simulink model "Robot_simulation"  (R2025b)
settings: Solver=VariableStepAuto  StartTime=0.0  StopTime=10  FixedStep=dt  RelTol=1e-3
InitFcn:
  | run("init.m");
values from neighbouring files (symbols this model uses):
  dt = 0.01    [init.m]
  F_max = 1500    [init.m]
  F_min = 100    [init.m]
  g = 9.81    [init.m]
  k_d = diag([5000, 5000])    [init.m]
  k_p = diag([20000, 20000])    [init.m]
  L_max = 0.8    [init.m]
  m3 = 60    [init.m]
  mb = 73    [init.m]
  mu = 0.6    [init.m]
  N = 15    [init.m]
  q_init = cinematica_inversa_2R(0, 0.6, robot_params)    [init.m]
  S_bar = 10*kron(eye(N), S)    [init.m]
  W_bar = kron(eye(N), W)    [init.m]
  x_ref = zeros(4, steps)    [init.m]
  x_ref_global = x_ref    [init.m]
  zb = 0.6    [init.m]
undefined symbols (not defined in the file or in its folder): DiscIntNeverNeededParam, robot_params
settings Model: Creator=Acer  LastModifiedBy=Acer

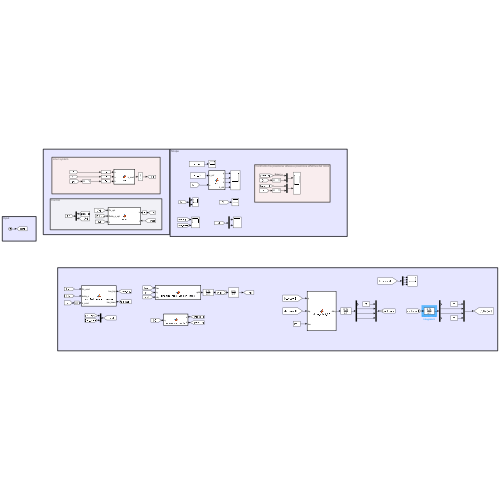
[thumbnail: Simulink's stored preview of the top-level diagram]
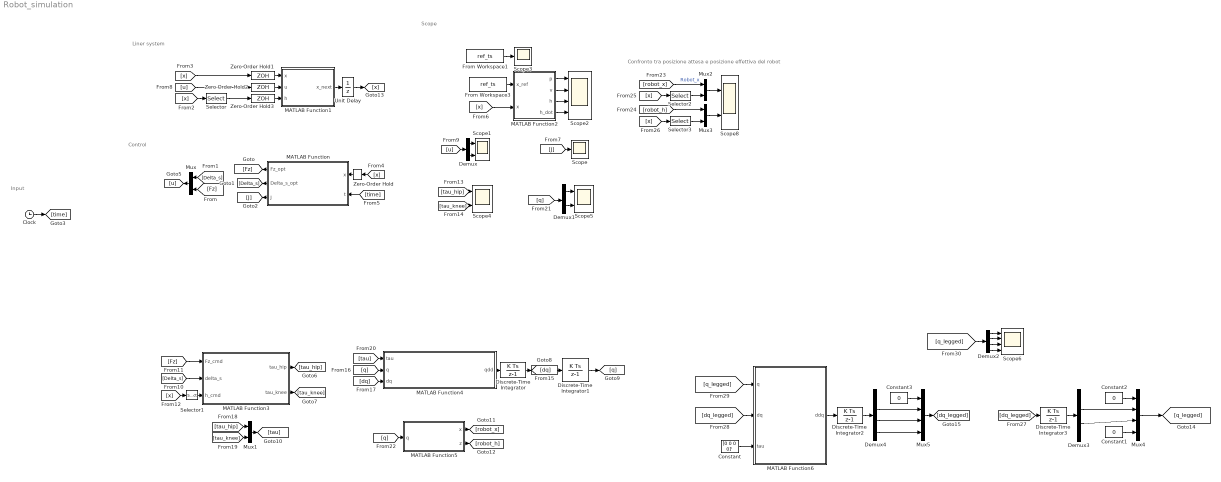
== system Robot_simulation ==
  note: Confronto tra posizione attesa e posizione effettiva del robot
  note: Control
  note: Liner system
  note: Input
  note: Scope
  Clock : Clock
  Constant : Constant  Value=[0 0 0 0]'
  Constant1 : Constant  Value=0
  Constant2 : Constant  Value=0
  Constant3 : Constant  Value=0
  Demux : Demux  Outputs=2
  Demux1 : Demux  Outputs=2
  Demux2 : Demux
  Demux3 : Demux
  Demux4 : Demux
  Discrete-Time Integrator : DiscreteIntegrator  InitialCondition=[0;0]  SampleTime=dt  ICPrevOutput=DiscIntNeverNeededParam  ICPrevScaledInput=DiscIntNeverNeededParam
  Discrete-Time Integrator1 : DiscreteIntegrator  InitialCondition=q_init  SampleTime=dt  ICPrevOutput=DiscIntNeverNeededParam  ICPrevScaledInput=DiscIntNeverNeededParam
  Discrete-Time Integrator2 : DiscreteIntegrator  InitialCondition=[0;0;0;0]  SampleTime=dt  ICPrevOutput=DiscIntNeverNeededParam  ICPrevScaledInput=DiscIntNeverNeededParam
  Discrete-Time Integrator3 : DiscreteIntegrator  InitialCondition=[0;-pi/2;0;0]  SampleTime=dt  ICPrevOutput=DiscIntNeverNeededParam  ICPrevScaledInput=DiscIntNeverNeededParam
  From Workspace1 : FromWorkspace  VariableName=ref_ts
  From Workspace3 : FromWorkspace  VariableName=ref_ts
  MATLAB Function : MATLAB Function  TreatAsAtomicUnit=on
  MATLAB Function1 : MATLAB Function  TreatAsAtomicUnit=on
  MATLAB Function2 : MATLAB Function  TreatAsAtomicUnit=on
  MATLAB Function3 : MATLAB Function  TreatAsAtomicUnit=on
  MATLAB Function4 : MATLAB Function  TreatAsAtomicUnit=on
  MATLAB Function5 : MATLAB Function  TreatAsAtomicUnit=on
  MATLAB Function6 : MATLAB Function  TreatAsAtomicUnit=on
  Mux{,1..3} (4 alike) : Mux  Inputs=2
  Mux4 : Mux
  Mux5 : Mux
  Scope : Scope
      settings: ActiveDisplayYMinimum=-1  ActiveDisplayYMaximum=1
  Scope{1,4..5,8} (4 alike) : Scope  NumInputPorts=2
      Scope1 settings: ActiveDisplayYMinimum=-0.020895768490500677  ActiveDisplayYMaximum=0.022328941684971165
      Scope4 settings: ActiveDisplayYMinimum=-14.847421541103996  ActiveDisplayYMaximum=15.870341136845298  DataLoggingVariableName=ScopeData4
      Scope5 settings: ActiveDisplayYMinimum=-1.7751159329900787E+253  ActiveDisplayYMaximum=1.5976043396910712E+254  DataLoggingVariableName=ScopeData5
      Scope8 settings: ActiveDisplayYMinimum=-0.36217276540062449  ActiveDisplayYMaximum=0.70314129266158121  DataLoggingVariableName=ScopeData8
  Scope2 : Scope  NumInputPorts=4
      settings: ActiveDisplayYMinimum=-0.12506830722069195  ActiveDisplayYMaximum=1.1256147649862278  DataLoggingVariableName=ScopeData2
  Scope3 : Scope
      settings: ActiveDisplayYMinimum=-1  ActiveDisplayYMaximum=1  DataLoggingVariableName=ScopeData3
  Scope6 : Scope  NumInputPorts=4
      settings: ActiveDisplayYMinimum=-1  ActiveDisplayYMaximum=1  DataLoggingVariableName=ScopeData6
  Selector : Selector  InputPortWidth=4  IndexOptions=Index vector (dialog)  Indices=[3]  OutputSizes=1
  Selector1 : Selector  InputPortWidth=4  IndexOptions=Index vector (dialog)  Indices=[3]  OutputSizes=1
  Selector2 : Selector  InputPortWidth=4  IndexOptions=Index vector (dialog)  Indices=1  OutputSizes=1
  Selector3 : Selector  InputPortWidth=4  IndexOptions=Index vector (dialog)  Indices=[3]  OutputSizes=1
  Unit Delay : UnitDelay  InitialCondition=x_ref(:,1)  SampleTime=-1  HasFrameUpgradeWarning=on
  Zero-Order Hold{,1..3} (4 alike) : ZeroOrderHold  SampleTime=dt
  wires:
  From Workspace1/1 -> Scope3/1
  MATLAB Function1/1(x_next) -> Unit Delay/1
  MATLAB Function/1(Fz_opt) -> [Fz]
  MATLAB Function/2(Delta_s_opt) -> [Delta_s]
  MATLAB Function/3(J) -> [J]
  Clock/1 -> [time]
  Unit Delay/1 -> [x]
  [Delta_s] -> Mux/1
  [Fz] -> Mux/2
  [x] -> Selector/1
  From Workspace3/1 -> MATLAB Function2/1(x_ref)
  MATLAB Function2/2(v) -> Scope2/2
  MATLAB Function2/1(p) -> Scope2/1
  MATLAB Function2/3(h) -> Scope2/3
  MATLAB Function2/4(h_dot) -> Scope2/4
  [x] -> MATLAB Function2/2(x)
  [J] -> Scope/1
  Mux/1 -> [u]
  [u] -> Demux/1
  Demux/1 -> Scope1/1
  Demux/2 -> Scope1/2
  [Delta_s] -> MATLAB Function3/2(delta_s)
  [Fz] -> MATLAB Function3/1(Fz_cmd)
  [x] -> Selector1/1
  Selector1/1 -> MATLAB Function3/3(h_cmd)
  MATLAB Function3/1(tau_hip) -> [tau_hip]
  MATLAB Function3/2(tau_knee) -> [tau_knee]
  [tau_knee] -> Scope4/2
  [tau_hip] -> Scope4/1
  MATLAB Function4/1(qdd) -> Discrete-Time Integrator/1
  Discrete-Time Integrator/1 -> [dq]
  [dq] -> Discrete-Time Integrator1/1
  Discrete-Time Integrator1/1 -> [q]
  [q] -> MATLAB Function4/2(q)
  [dq] -> MATLAB Function4/3(dq)
  [tau_hip] -> Mux1/1
  [tau_knee] -> Mux1/2
  Mux1/1 -> [tau]
  [tau] -> MATLAB Function4/1(tau)
  [q] -> Demux1/1
  Demux1/1 -> Scope5/1
  Demux1/2 -> Scope5/2
  MATLAB Function5/1(x) -> [robot_x]
  MATLAB Function5/2(z) -> [robot_h]
  [q] -> MATLAB Function5/1(q)
  [x] -> Selector2/1
  [x] -> Selector3/1
  [robot_x] -> Mux2/1  "Robot_x"
  Selector2/1 -> Mux2/2
  [robot_h] -> Mux3/1
  Selector3/1 -> Mux3/2
  Mux2/1 -> Scope8/1
  Mux3/1 -> Scope8/2
  Zero-Order Hold/1 -> MATLAB Function/1(x)
  [x] -> Zero-Order Hold/1
  [time] -> MATLAB Function/2(t)
  Constant/1 -> MATLAB Function6/3(tau)
  MATLAB Function6/1(ddq) -> Discrete-Time Integrator2/1
  [dq_legged] -> Discrete-Time Integrator3/1
  [q_legged] -> MATLAB Function6/1(q)
  Demux2/1 -> Scope6/1
  Demux2/2 -> Scope6/2
  Demux2/3 -> Scope6/3
  Demux2/4 -> Scope6/4
  [x] -> Zero-Order Hold1/1
  Zero-Order Hold1/1 -> MATLAB Function1/1(x)
  [u] -> Zero-Order Hold2/1
  Zero-Order Hold2/1 -> MATLAB Function1/2(u)
  Selector/1 -> Zero-Order Hold3/1
  Zero-Order Hold3/1 -> MATLAB Function1/3(h)
  [dq_legged] -> MATLAB Function6/2(dq)
  [q_legged] -> Demux2/1
  Constant1/1 -> Mux4/4
  Constant2/1 -> Mux4/1
  Discrete-Time Integrator3/1 -> Demux3/1
  Demux3/2 -> Mux4/2
  Demux3/3 -> Mux4/3
  Mux4/1 -> [q_legged]
  Discrete-Time Integrator2/1 -> Demux4/1
  Mux5/1 -> [dq_legged]
  Demux4/3 -> Mux5/3
  Constant3/1 -> Mux5/1
  Demux4/2 -> Mux5/2
  Demux4/4 -> Mux5/4

== matlab function Robot_simulation/MATLAB Function6 ==
  data: q input; ddq output size=4; dq input; tau input
function ddq =  whole_robot_2D(q, dq, tau)
    % tau è il vettore delle coppie/forze generalizzate in ingresso (4x1)
    
    % 1. Calcola le matrici dinamiche valutate nello stato attuale
    [M, C, G] = Dinamica_Robot(q, dq);
    
    % 2. Risolvi l'equazione del moto: M*ddq + C*dq + G = tau
    % In MATLAB/Simulink si usa l'operatore mldivide (\) per invertire M in modo robusto
    ddq = M \ (tau - C*dq - G);
end

== matlab function Robot_simulation/MATLAB Function1 ==
  data: x input size=4; x_next output size=4; u input size=2; h input size=1; g parameter; mb parameter; dt parameter
function x_next = fcn(x,u,h,g, mb,dt)

dc = [0; 0; 0; -g];     % Disturbo di gravità
dk = dc * dt;

Ac = [0 1 0 0; 0 0 0 0; 0 0 0 1; 0 0 0 0];
Bc = [0 0; g/h 0; 0 0; 0 1/mb];

    Ak = eye(4) + Ac * dt;
    Bk = Bc * dt;

   %dk disturbo di gravita
x_next = Ak*x + Bk*u + dk;

== matlab function Robot_simulation/MATLAB Function ==
  data: x input; Fz_opt output; t input; Delta_s_opt output; J output; zb parameter; g parameter; m3 parameter; dt parameter; mu parameter; W_bar parameter; S_bar parameter; F_max parameter; F_min parameter; N parameter; L_max parameter; x_ref_global parameter
function [Fz_opt, Delta_s_opt, J] = MPC(x,t,...              %INPUT
                                    zb, g, m3, dt, mu, W_bar, S_bar, F_max, F_min, N, L_max, x_ref_global) %PARAMETERS
% INPUT:
    % x_ref_global: Matrice intera della traiettoria [4 x steps]
    % t: Tempo di simulazione attuale (da un blocco Clock)

    % --- 1. GESTIONE DELLA TRAIETTORIA (SLIDING WINDOW) ---
    steps_totali = size(x_ref_global, 2);
    
    % Calcolo dell'indice attuale k basato sul tempo
    % Aggiungiamo 1 perché MATLAB usa indici che partono da 1 (t=0 -> k=1)
    k_curr = floor(t / dt) + 1; 
    
    % Inizializza il vettore per l'orizzonte N
    X_ref_window = zeros(4*N, 1);
    
    for i = 1:N
        % Calcola l'indice futuro. Il "min" serve come saturazione: 
        % se l'orizzonte guarda oltre la fine della simulazione, tiene l'ultimo target.
        idx = min(k_curr + i - 1, steps_totali); 
        
        % Inserisce i 4 stati futuri nello slot corretto
        X_ref_window((i-1)*4+1 : i*4) = x_ref_global(:, idx);
    end
    

    % INPUT: 
    % x_ref DEVE essere un vettore colonna [4*N x 1]. Se è una matrice, 
    % devi srotolarla prima di questa riga.

    h_k = x(3);
    dc = [0; 0; 0; -g];     % Disturbo di gravità
    dk = dc * dt;
    
    % --- Ricalcolo Dinamica Locale basata su h_k ---
    Ac = [0 1 0 0; 0 0 0 0; 0 0 0 1; 0 0 0 0];
    Bc = [0 0; g/h_k 0; 0 0; 0 1/m3];
    Ak = eye(4) + Ac * dt;
    Bk = Bc * dt;
    
    % --- Aggiornamento Dinamico dei Vincoli ---
    max_kinematic_ds = sqrt(L_max^2 - zb^2);
    ds_min = max(-mu*h_k, -max_kinematic_ds);
    ds_max = min(mu*h_k, max_kinematic_ds);
    
    U_min = [ds_min; F_min];
    U_max = [ds_max; F_max];
    LB = repmat(U_min, N, 1);
    UB = repmat(U_max, N, 1);
    
    % --- Calcolo Matrici di Predizione per l'orizzonte N ---
    Phi = zeros(4*N, 2*N);
    Psi = zeros(4*N, 4);
    Term_dist = zeros(4*N, 1);
    
    for i = 1:N
        Psi((i-1)*4+1:i*4, :) = Ak^i;
        for j = 1:i
            Phi((i-1)*4+1:i*4, (j-1)*2+1:j*2) = (Ak^(i-j)) * Bk;
            Term_dist((i-1)*4+1:i*4) = Term_dist((i-1)*4+1:i*4) + (Ak^(i-j))*dk;
        end
    end
    
    H = 2 * (Phi' * S_bar * Phi + W_bar);
    f = 2 * Phi' * S_bar * (Psi * x + Term_dist - X_ref_window);

 % --- 5. RISOLUZIONE QP ---
    options = optimoptions('quadprog', 'Algorithm', 'active-set', 'Display', 'off');
    
    % Definisci l'ingresso di equilibrio (Delta_s = 0, F_z = massa * gravità)
    u_guess_step = [0; m3* g];
    
    % Replicato per tutto l'orizzonte N
    U0_guess = repmat(u_guess_step, N, 1);
    
    % Passa U0_guess come 9° argomento invece di []
    [U_seq, fval, exitflag] = quadprog(H, f, [], [], [], [], LB, UB,U0_guess,options);
    
    % % --- Failsafe: Protezione contro il crash del solver ---
    % if exitflag <= 0 || isempty(U_seq)
    %     % Se fallisce, forza gli input a zero o a un valore di sicurezza
    %     U_seq = zeros(2*N, 1);
    %     fval = 0;
    % end
    
    % --- Calcolo del vero costo ---
    Errore_non_controllato = (Psi * x + Term_dist - X_ref_window);
    cost_costante = Errore_non_controllato' * S_bar * Errore_non_controllato;
    J = fval + cost_costante;
    
    % --- Assegnazione Output Corretta ---
    u_opt = U_seq(1:2);
    Delta_s_opt = u_opt(1); % u_1 controlla la dinamica x
    Fz_opt = u_opt(2);      % u_2 controlla la dinamica z

end

== matlab function Robot_simulation/MATLAB Function2 ==
  data: x_ref input; p output; x input; v output; h output; h_dot output
function [p, v, h, h_dot] = fcn(x_ref,x)

p = [x_ref(1),x(1)];
v = [x_ref(2),x(2)];
h = [x_ref(3),x(3)];
h_dot = [x_ref(4),x(4)];

== matlab function Robot_simulation/MATLAB Function3 ==
  data: Fz_cmd input; tau_hip output; delta_s input; h_cmd input; k_p parameter; k_d parameter; tau_knee output; robot_params parameter
function [tau_hip, tau_knee] = new_Task_space_controller(Fz_cmd, delta_s, h_cmd, k_p, k_d, robot_params)
    %% 1. Cinematica Inversa (IK) - Modello D-H Standard
    % Target: [delta_s; h_cmd] (posizione end-effector)
    % L'ipotenusa L

    l1 = robot_params.l1;
    l2 = robot_params.l2;

    dist_sq = delta_s^2 + h_cmd^2;
    L = sqrt(dist_sq);
    
    % Legge del coseno per q2 (relativo)
    cos_q2 = (dist_sq - l1^2 - l2^2) / (2 * l1 * l2);
    cos_q2 = max(min(cos_q2, 1), -1); % Saturazione numerica
    q2 = acos(cos_q2); % Configurazione: ginocchio flesso positivo
    
    % Angolo q1 (anca)
    q1 = atan2(h_cmd, delta_s) - atan2(l2*sin(q2), l1 + l2*cos(q2));
    
    %% 2. Jacobiano Analitico (D-H Standard)
    % J = [dx/dq1, dx/dq2; dy/dq1, dy/dq2]
    s1 = sin(q1); c1 = cos(q1);
    s12 = sin(q1 + q2); c12 = cos(q1 + q2);
    
    J = [ -l1*s1 - l2*s12, -l2*s12;
           l1*c1 + l2*c12,  l2*c12 ];
         
    %% 3. VIRTUAL MODEL CONTROL
    % Posizione end-effector calcolata dalla cinematica diretta (D-H)
    x_e = l1*c1 + l2*c12;
    y_e = l1*s1 + l2*s12;
    p_f = [x_e; y_e];
    p_d = [delta_s; h_cmd];
    
    % Velocità (assumiamo 0 per semplicità, ma andrebbero lette dai giunti)
    v_f = [0; 0];
    v_d = [0; 0];
    
    % Forza di controllo nel Task Space
    F_feedback = k_p * (p_d - p_f) + k_d * (v_d - v_f);
    F_feedforward = [0; Fz_cmd]; 
    F_tot = F_feedback + F_feedforward;
    
    %% 4. Mapping delle coppie (J' * F)
    % La trasposta dello Jacobiano mappa le forze cartesiane nelle coppie ai giunti
    Tau = J' * F_tot;
    
    % Assegnazione corretta: 
    % Tau(1) -> Giunto 1 (Hip), Tau(2) -> Giunto 2 (Knee)
    tau_hip  = Tau(1); 
    tau_knee = Tau(2); 
end

== matlab function Robot_simulation/MATLAB Function4 ==
  data: tau input; q input; qdd output; dq input; robot_params parameter; g parameter
function qdd   = dinamica_robot_2R_con_carico(tau, q, dq, robot_params, g)
    % Carico applicato sull'end effector (kg)
    mL = 60; 

    % Estrazione variabili di stato
    theta1 = q(1);
    theta2 = q(2);
    dtheta1 = dq(1);
    dtheta2 = dq(2);

    % Estrazione parametri corretti per il 2R
    m1 = robot_params.m1;   
    m2 = robot_params.m2;
    l1 = robot_params.l1;   
    l2 = robot_params.l2;
    lc1 = robot_params.lc1; 
    lc2 = robot_params.lc2;
    I1 = robot_params.I1;   
    I2 = robot_params.I2;


    % 1. Matrice di Inerzia B(q)
    b11 = m1*lc1^2 + I1 + m2*(l1^2 + lc2^2 + 2*l1*lc2*cos(theta2)) + I2 + ...
          mL*(l1^2 + l2^2 + 2*l1*l2*cos(theta2));
    b12 = m2*(lc2^2 + l1*lc2*cos(theta2)) + I2 + ...
          mL*(l2^2 + l1*l2*cos(theta2));
    b21 = b12; 
    b22 = m2*lc2^2 + I2 + mL*l2^2;
    B = [b11, b12; b21, b22];

    % 2. Matrice di Coriolis e forze centrifughe C(q, dq)
    h = (m2*lc2 + mL*l2) * l1 * sin(theta2);
    c11 = -h * dtheta2;
    c12 = -h * (dtheta1 + dtheta2);
    c21 =  h * dtheta1;
    c22 =  0;
    C = [c11, c12; c21, c22];

    % 3. Vettore di Gravità G(q)
    g1 = (m1*lc1 + m2*l1 + mL*l1) * g * cos(theta1) + ...
         (m2*lc2 + mL*l2) * g * cos(theta1 + theta2);
    g2 = (m2*lc2 + mL*l2) * g * cos(theta1 + theta2);
    G = [g1; g2];

    qdd = B\ (tau - C*dq - G );
end

== matlab function Robot_simulation/MATLAB Function5 ==
  data: q input; x output; z output; robot_params parameter
function [x,z] = cinematica_diretta(q,robot_params)


[x,z] = cinematica_diretta_2R(q, robot_params);
